simulink model "Block_fixedQ_Ccode_expanded"  (R2017b)
settings: Solver=VariableStepAuto  StartTime=0.0  StopTime=Test_time  RelTol=1e-3
values from neighbouring files (symbols this model uses):
  Lq = length(F.Omega(:,:,1))    [Saveconstraints.m]
  Ts = plant.Ts    [CoprimeFactorizationSS.m]    (also in ID_Model.m = 0.001; ID_Model_4.m = 0.001; ID_Model_ITRI.m = 0.001; gConstraintFun.m = P.Ts)
  Vmax = 300    [ID_Model.m]    (also in ID_Model_4.m; ID_Model_ITRI.m)
undefined symbols (not defined in the file or in its folder): plant, Qnum
settings Model: Creator=LAB_JHU  LastModifiedBy=Johnny

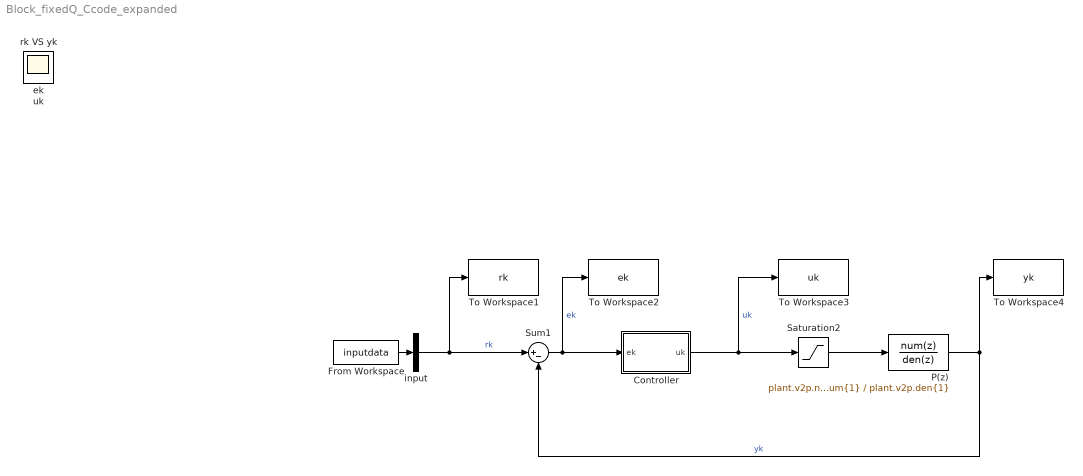
== system Block_fixedQ_Ccode_expanded ==
  Controller : Subsystem
  From Workspace : FromWorkspace  VariableName=inputdata  SampleTime=Ts
  P(z) : DiscreteTransferFcn  Numerator=plant.v2p.num{1}  Denominator=plant.v2p.den{1}  SampleTime=Ts
  Saturation2 : Saturate  UpperLimit=Vmax  LowerLimit=-Vmax
  Sum1 : Sum  Inputs=|+-
  To Workspace1 : ToWorkspace  VariableName=rk  SampleTime=-1
  To Workspace2 : ToWorkspace  VariableName=ek  SampleTime=-1
  To Workspace3 : ToWorkspace  VariableName=uk  SampleTime=-1
  To Workspace4 : ToWorkspace  VariableName=yk  SampleTime=-1
  input : Demux  Outputs=1
  ek : Scope
  rk VS yk : Scope
  uk : Scope
  wires:
  Saturation2/1 -> P(z)/1
  Sum1/1 -> To Workspace2/1, Controller/1(ek)  "ek"
  P(z)/1 -> To Workspace4/1, Sum1/2  "yk"
  Controller/1(uk) -> To Workspace3/1, Saturation2/1  "uk"
  input/1 -> Sum1/1, To Workspace1/1  "rk"
  From Workspace/1 -> input/1

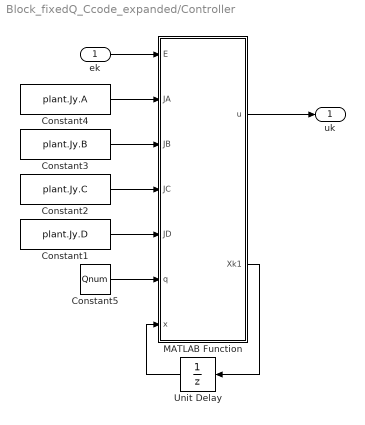
== system Block_fixedQ_Ccode_expanded/Controller ==
  ek : Inport
  Constant1 : Constant  Value=plant.Jy.D
  Constant2 : Constant  Value=plant.Jy.C
  Constant3 : Constant  Value=plant.Jy.B
  Constant4 : Constant  Value=plant.Jy.A
  Constant5 : Constant  Value=Qnum
  MATLAB Function : MATLAB Function  TreatAsAtomicUnit=on
  Unit Delay : UnitDelay  InitialCondition=zeros(Lq+4,1)  SampleTime=-1
  uk : Outport
  wires:
  Constant5/1 -> MATLAB Function/6(q)
  Unit Delay/1 -> MATLAB Function/7(x)
  MATLAB Function/2(Xk1) -> Unit Delay/1
  MATLAB Function/1(u) -> uk/1
  ek/1 -> MATLAB Function/1(E)
  Constant4/1 -> MATLAB Function/2(JA)
  Constant3/1 -> MATLAB Function/3(JB)
  Constant2/1 -> MATLAB Function/4(JC)
  Constant1/1 -> MATLAB Function/5(JD)

== matlab function Block_fixedQ_Ccode_expanded/Controller/MATLAB Function ==
  data: E input; JA input; JB input; JC input; JD input; q input; u output; x input; Xk1 output
function [u,Xk1] = C_expanded(E,JA,JB,JC,JD,q,x)

q0 = q(1);
qxsum = q(2:length(q)).'*x(6:length(x));

% % general
X0 = (JA(1,:)+JB(1,2)*q0*JC(2,:))*x(1:5) + E*(JB(1,1)+JB(1,2)*JD(2,1)*q0) + JB(1,2)*qxsum;

X1 = (JA(2,:)+JB(2,2)*q0*JC(2,:))*x(1:5) + E*(JB(2,1)+JB(2,2)*JD(2,1)*q0) + JB(2,2)*qxsum;

X2 = (JA(3,:)+JB(3,2)*q0*JC(2,:))*x(1:5) + E*(JB(3,1)+JB(3,2)*JD(2,1)*q0) + JB(3,2)*qxsum;

X3 = (JA(4,:)+JB(4,2)*q0*JC(2,:))*x(1:5) + E*(JB(4,1)+JB(4,2)*JD(2,1)*q0) + JB(4,2)*qxsum;   

X4 = (JA(5,:)+JB(5,2)*q0*JC(2,:))*x(1:5) + E*(JB(5,1)+JB(5,2)*JD(2,1)*q0) + JB(5,2)*qxsum;

Z0 = JD(2,1)*E + JC(2,:)*x(1:5);

Z = x(6:length(x)-1);

Xk1 = [X0; X1; X2; X3; X4; Z0; reshape(Z,[length(Z),1])];

u = (JC(1,:)+q0*JC(2,:)*JD(1,2))*x(1:5) + JD(1,2)*JD(2,1)*E*q0 + JD(1,2)*qxsum;

end
